simulink library "RobotX_Lib"  (R2015b)
settings: Solver=VariableStepAuto  StartTime=0.0  StopTime=10.0  RelTol=1e-3
settings Model: Creator=jorgemartins  LastModifiedBy=jorgemartins

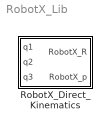
== system RobotX_Lib ==
  RobotX_Direct_Kinematics : MATLAB Function  TreatAsAtomicUnit=on

== matlab function RobotX_Lib/RobotX_Direct_Kinematics ==
  data: q1 input; RobotX_R output; q2 input; q3 input; RobotX_p output
function [RobotX_R,RobotX_p] = RobotX_Direct_Kinematics(q1,q2,q3)
%#codegen

%    This function was generated by the Symbolic Math Toolbox version 6.3.
%    10-Mar-2016 14:49:48

t2 = cos(q1);
t3 = sin(q1);
t4 = sin(q2);
t5 = cos(q2);
RobotX_R = reshape([-t2.*t4,-t3.*t4,t5,t3,-t2,0.0,t2.*t5,t3.*t5,t4],[3,3]);
if nargout > 1
    t6 = q3.*t5.*2.0;
    t7 = -t4+t5+t6;
    RobotX_p = [t2.*t7.*(1.0./2.0);t3.*t7.*(1.0./2.0);t4.*(1.0./2.0)+t5.*(1.0./2.0)+q3.*t4];
end
